simulink model "TurnLights_System_Model"  (R2024b)
settings: Solver=VariableStepAuto  StartTime=0.0  StopTime=45  RelTol=1e-3
settings Model: PacingRate=0.790000  Creator=pjman  LastModifiedBy=pjman
settings OptimizationCC: DefaultParameterBehavior=Inlined  EnhancedBackFolding=on  PassReuseOutputArgsAs=Individual arguments  ZeroExternalMemoryAtStartup=off  ZeroInternalMemoryAtStartup=off  OptimizeBlockOrder=speed  DifferentSizesBufferReuse=on  OptimizationCustomize=off  EfficientTunableParamExpr=on
settings DebuggingCC: ParameterTunabilityLossMsg=error  BusObjectLabelMismatch=error
settings SFSimCC: MATLABDynamicMemAlloc=off
settings RTWCC: Description=Embedded Coder  SystemTargetFile=ert.tlc  TemplateMakefile=ert_default_tmf
settings CodeAppCC: ForceParamTrailComments=on  IgnoreCustomStorageClasses=off  OperatorAnnotations=on  SimulinkDataObjDesc=on  SFDataObjDesc=on  InsertBlockDesc=on
settings ERTTargetCC: TargetLangStandard=C99 (ISO)  GenerateSampleERTMain=on  ERTCustomFileTemplate=example_file_process.tlc

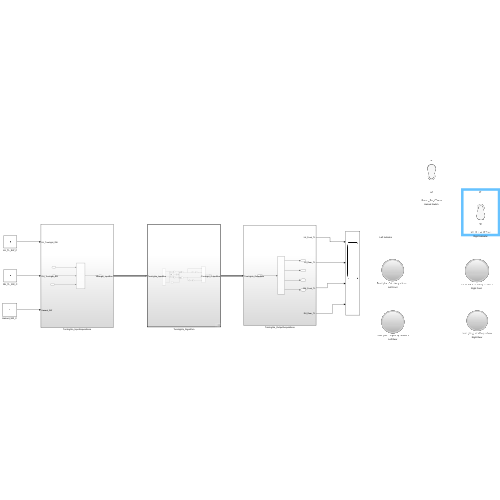
[thumbnail: Simulink's stored preview of the top-level diagram]
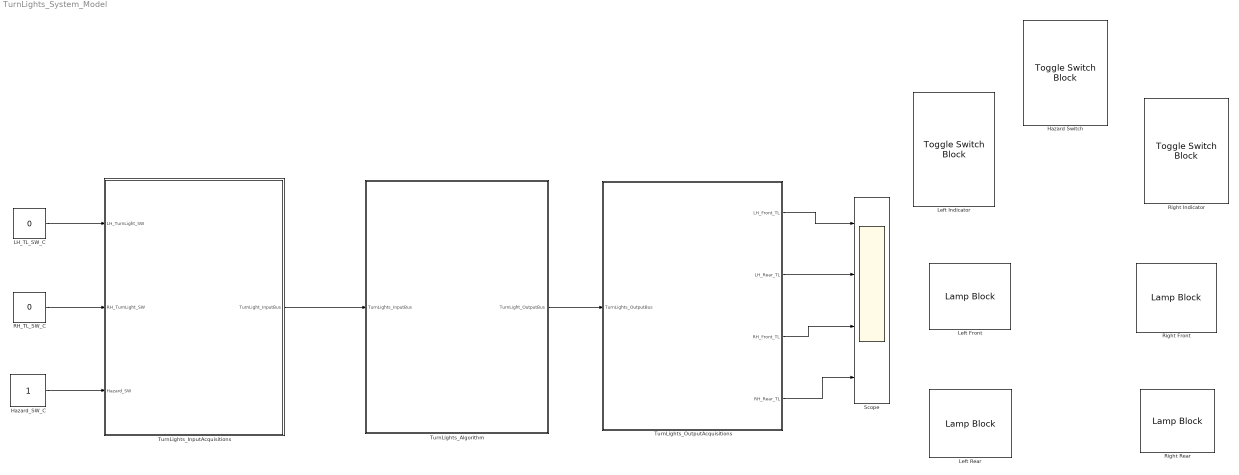
== system TurnLights_System_Model ==
  Hazard Switch : ToggleSwitchBlock  LabelPosition=Bottom
      settings: Values={{'Off', 'On'}, [0 1]}
  Hazard_SW_C : Constant  OutDataTypeStr=boolean
  LH_TL_SW_C : Constant  Value=0  OutDataTypeStr=boolean
  Left Front : LampBlock  LabelPosition=Bottom
  "Left Indicator " : ToggleSwitchBlock  LabelPosition=Bottom
      settings: Values={{'Off', 'On'}, [0 1]}
  Left Rear : LampBlock  LabelPosition=Bottom
  RH_TL_SW_C : Constant  Value=0  OutDataTypeStr=boolean
  Right Front : LampBlock  LabelPosition=Bottom
  Right Indicator : ToggleSwitchBlock  LabelPosition=Bottom
      settings: Values={{'Off', 'On'}, [0 1]}
  Right Rear : LampBlock  LabelPosition=Bottom
  Scope : Scope  NumInputPorts=4
  TurnLights_Algorithm : Subsystem  TreatAsAtomicUnit=on
  TurnLights_InputAcquisitions : Subsystem
  TurnLights_OutputAcquisitions : Subsystem
  wires:
  LH_TL_SW_C/1 -> TurnLights_InputAcquisitions/1(LH_TurnLight_SW)
  RH_TL_SW_C/1 -> TurnLights_InputAcquisitions/2(RH_TurnLight_SW)
  Hazard_SW_C/1 -> TurnLights_InputAcquisitions/3(Hazard_SW)
  TurnLights_InputAcquisitions/1(TurnLight_InputBus) -> TurnLights_Algorithm/1(TurnLights_InputBus)
  TurnLights_Algorithm/1(TurnLight_OutputBus) -> TurnLights_OutputAcquisitions/1(TurnLights_OutputBus)
  TurnLights_OutputAcquisitions/1(LH_Front_TL) -> Scope/1
  TurnLights_OutputAcquisitions/2(LH_Rear_TL) -> Scope/2
  TurnLights_OutputAcquisitions/4(RH_Rear_TL) -> Scope/4
  TurnLights_OutputAcquisitions/3(RH_Front_TL) -> Scope/3

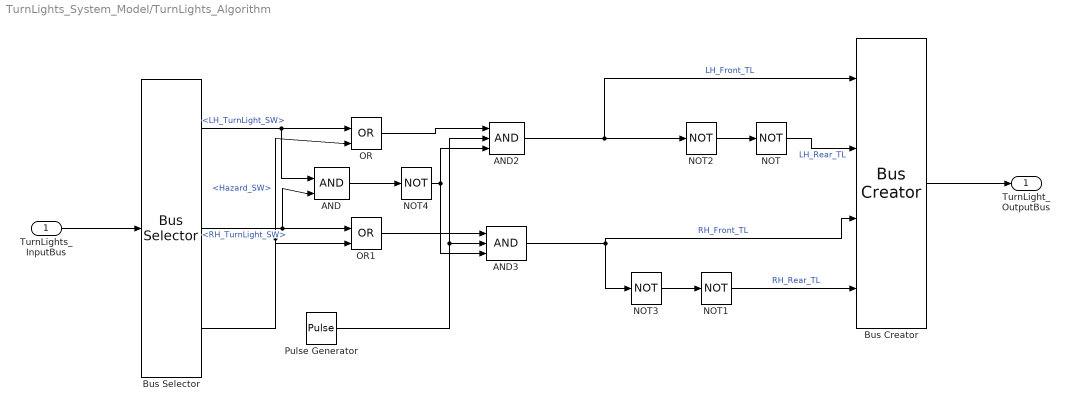
== system TurnLights_System_Model/TurnLights_Algorithm ==
  TurnLights_InputBus : Inport  OutDataTypeStr=Bus: TurnLights_InputBus
  AND : Logic  IconShape=distinctive  AllPortsSameDT=off  OutDataTypeStr=boolean
  AND2 : Logic  Inputs=3  IconShape=distinctive  AllPortsSameDT=off  OutDataTypeStr=boolean
  AND3 : Logic  Inputs=3  IconShape=distinctive  AllPortsSameDT=off  OutDataTypeStr=boolean
  Bus Creator : BusCreator  Inputs=4  OutDataTypeStr=Bus: TurnLights_OutputBus
  Bus Selector : BusSelector  OutputSignals=LH_TurnLight_SW,RH_TurnLight_SW,Hazard_SW
  NOT{,1..4} (5 alike) : Logic  Operator=NOT  IconShape=distinctive  AllPortsSameDT=off  OutDataTypeStr=boolean
  OR : Logic  Operator=OR  IconShape=distinctive  AllPortsSameDT=off  OutDataTypeStr=boolean
  OR1 : Logic  Operator=OR  IconShape=distinctive  AllPortsSameDT=off  OutDataTypeStr=boolean
  Pulse Generator : DiscretePulseGenerator  PulseType=Time based  PulseWidth=50
  TurnLight_OutputBus : Outport  OutDataTypeStr=Bus: TurnLights_OutputBus
  wires:
  TurnLights_InputBus/1 -> Bus Selector/1
  Bus Selector/1 -> AND/1, OR/1  "<LH_TurnLight_SW>"
  Bus Selector/2 -> AND/2, OR1/1  "<RH_TurnLight_SW>"
  Bus Selector/3 -> OR1/2, OR/2  "<Hazard_SW>"
  Pulse Generator/1 -> AND2/2, AND3/2
  AND3/1 -> NOT3/1, Bus Creator/3  "RH_Front_TL"
  NOT/1 -> Bus Creator/2  "LH_Rear_TL"
  NOT2/1 -> NOT/1
  AND2/1 -> Bus Creator/1, NOT2/1  "LH_Front_TL"
  NOT1/1 -> Bus Creator/4  "RH_Rear_TL"
  NOT3/1 -> NOT1/1
  Bus Creator/1 -> TurnLight_OutputBus/1
  OR/1 -> AND2/1
  OR1/1 -> AND3/1
  AND/1 -> NOT4/1
  NOT4/1 -> AND2/3, AND3/3

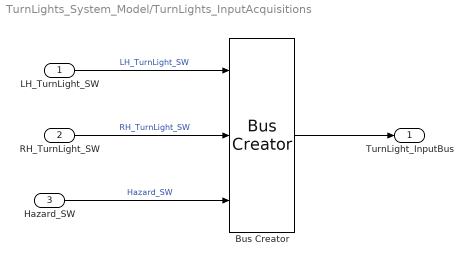
== system TurnLights_System_Model/TurnLights_InputAcquisitions ==
  LH_TurnLight_SW : Inport  OutDataTypeStr=boolean
  RH_TurnLight_SW : Inport  Port=2  OutDataTypeStr=boolean
  Hazard_SW : Inport  Port=3  OutDataTypeStr=boolean
  Bus Creator : BusCreator  Inputs=3  OutDataTypeStr=Bus: TurnLights_InputBus
  TurnLight_InputBus : Outport  OutDataTypeStr=Bus: TurnLights_InputBus
  wires:
  LH_TurnLight_SW/1 -> Bus Creator/1  "LH_TurnLight_SW"
  RH_TurnLight_SW/1 -> Bus Creator/2  "RH_TurnLight_SW"
  Hazard_SW/1 -> Bus Creator/3  "Hazard_SW"
  Bus Creator/1 -> TurnLight_InputBus/1

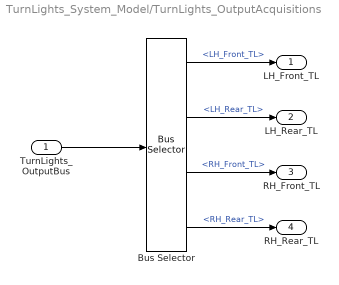
== system TurnLights_System_Model/TurnLights_OutputAcquisitions ==
  TurnLights_OutputBus : Inport  OutDataTypeStr=Bus: TurnLights_OutputBus
  Bus Selector : BusSelector  OutputSignals=LH_Front_TL,LH_Rear_TL,RH_Front_TL,RH_Rear_TL
  LH_Front_TL : Outport  OutDataTypeStr=boolean
  LH_Rear_TL : Outport  Port=2  OutDataTypeStr=boolean
  RH_Front_TL : Outport  Port=3  OutDataTypeStr=boolean
  RH_Rear_TL : Outport  Port=4  OutDataTypeStr=boolean
  wires:
  TurnLights_OutputBus/1 -> Bus Selector/1
  Bus Selector/1 -> LH_Front_TL/1  "<LH_Front_TL>"
  Bus Selector/2 -> LH_Rear_TL/1  "<LH_Rear_TL>"
  Bus Selector/3 -> RH_Front_TL/1  "<RH_Front_TL>"
  Bus Selector/4 -> RH_Rear_TL/1  "<RH_Rear_TL>"
